simulink model "State_Feedback_Osservatore_Integratore_R"  (R2024b)
settings: Solver=VariableStepAuto  StartTime=0.0  StopTime=ST  RelTol=1e-3
InitFcn:
  | % clear all
  | % close all
  | % clc
  | %
  | % % Load Modello e Parametri
  | % load("model.mat");
  | %
  | % load("Ass_autovalori.mat");
  | %
  | % double_A = double(A_lin);
  | % double_B = double(B_lin);
  | % C = [1 0 0 0 0 0; 0 0 1 0 0 0; 0 0 0 0 1 0];
  | % D = zeros(3,2);
  | % Kf = pinv(C*inv(A_closed_loop)*double_B);
  | %
  | % % Condizioni iniziali
  | % x0 = [1, 0, 0.44, 0, 0.03, 0]'; % Stato iniziale
  | %
  | % % Verifica dell'osservabilità
  | % O = obsv(A_lin, C); rank(O)
  | % osservabile = rank(O) == size(double_A, 1);
  | %
  | % if osservabile
  | %     disp('Il sistema è osservabile.');
  | % else
  | %     disp('Il sistema NON è osservabile.');
  | % end
  | %
  | % % Verifica dell'osservabilità
  | % Ctrb = ctrb(double_A', C');
  | % controllabile = rank(Ctrb) == size(double_A, 1);
  | %
  | % if controllabile
  | %     disp('Il sistema è controllabile.');
  | % else
  | %     disp('Il sistema NON è controllabile.');
  | % end
  | %
  | %
  | % % Poli desiderati per l'osservatore
  | % poli_osservatore = [-80 -2 -40 -1 -30 -0.5];
  | %
  | % % Calcolo del guadagno dell'osservatore L
  | % L = place(double_A', C', poli_osservatore)';
  | %
  | % % Dinamica dell'osservatore
  | % A_o = double_A - L * C; % Matrice del sistema osservatore
  | % B_o = [double_B - L * D, L]; % Matrice degli ingressi per l'osservatore
  | % C_o = eye(6); % Gli stati stimati vengono restituiti
  | % D_o = zeros(6,5); % Dimensioni appropriate per ingressi e uscite
undefined symbols (not defined in the file or in its folder): A_o, B_o, C, C_o, D, D_o, double_A, double_B, K_i, x0, x0_Aug, xd_aug
libraries: simulink x1
settings Model: Creator=raffa  LastModifiedBy=raffa
settings RTWCC: GPUComputeCapability=3.5

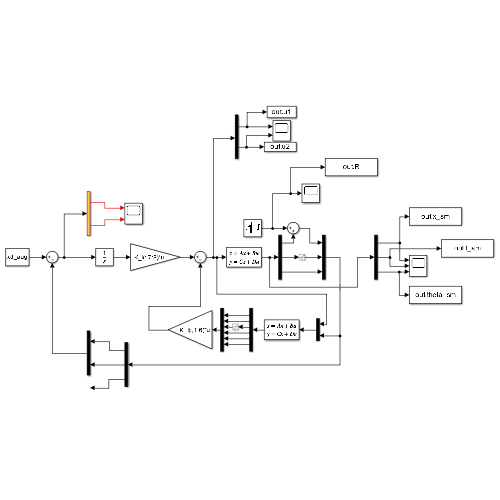
[thumbnail: Simulink's stored preview of the top-level diagram]
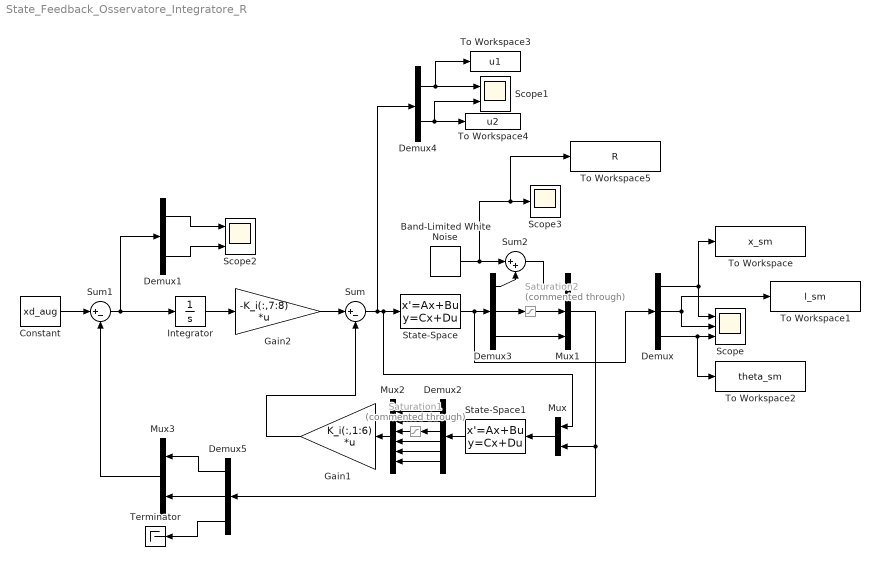
== system State_Feedback_Osservatore_Integratore_R ==
  Band-Limited White Noise : simulink/Sources/Band-Limited White Noise  Cov=[0.00005]  Ts=0.1  seed=[23341]
  Constant : Constant  Value=xd_aug
  Demux : Demux  Outputs=3
  Demux1 : Demux  Outputs=2
  Demux2 : Demux  Outputs=6
  Demux3 : Demux  Outputs=3
  Demux4 : Demux  Outputs=2
  Demux5 : Demux  Outputs=3
  Gain1 : Gain  Gain=K_i(:,1:6)  Multiplication=Matrix(K*u)
  Gain2 : Gain  Gain=-K_i(:,7:8)  Multiplication=Matrix(K*u)
  Integrator : Integrator  InitialCondition="[1 0 0 0 0 0 0 0; 0 0  1 0 0 0 0 0] * x0_Aug"
  Mux : Mux  Inputs=2
  Mux1 : Mux  Inputs=3
  Mux2 : Mux  Inputs=6
  Mux3 : Mux  Inputs=2
  Saturation1 : Saturate  Commented=through  UpperLimit=2  LowerLimit=0.1
  Saturation2 : Saturate  Commented=through  UpperLimit=2  LowerLimit=0.1
  Scope : Scope  NumInputPorts=3
  Scope1 : Scope  NumInputPorts=2
  Scope2 : Scope  NumInputPorts=2
  Scope3 : Scope
  State-Space : StateSpace  A=double_A  B=double_B  C=C  D=D  InitialCondition=x0
  State-Space1 : StateSpace  A=A_o  B=B_o  C=C_o  D=D_o  InitialCondition=x0
  Sum : Sum  Inputs=|+-
  Sum1 : Sum  Inputs=|+-
  Sum2 : Sum  Inputs=|++
  Terminator : Terminator
  To Workspace : ToWorkspace  VariableName=x_sm  SaveFormat=Timeseries  SampleTime=-1
  To Workspace1 : ToWorkspace  VariableName=l_sm  SaveFormat=Timeseries  SampleTime=-1
  To Workspace2 : ToWorkspace  VariableName=theta_sm  SaveFormat=Timeseries  SampleTime=-1
  To Workspace3 : ToWorkspace  VariableName=u1  SaveFormat=Timeseries  SampleTime=-1
  To Workspace4 : ToWorkspace  VariableName=u2  SaveFormat=Timeseries  SampleTime=-1
  To Workspace5 : ToWorkspace  VariableName=R  SaveFormat=Timeseries  SampleTime=-1
  wires:
  Mux1/1 -> Demux5/1, Mux/2
  Gain1/1 -> Sum/2
  Demux/1 -> Scope/1, To Workspace/1
  Demux/2 -> Scope/2, To Workspace1/1
  Mux/1 -> State-Space1/1
  Integrator/1 -> Gain2/1
  Constant/1 -> Sum1/1
  Gain2/1 -> Sum/1
  Sum1/1 -> Integrator/1, Demux1/1
  Demux1/1 -> Scope2/1
  Demux2/1 -> Mux2/1
  Demux2/2 -> Mux2/2
  State-Space1/1 -> Demux2/1
  Mux2/1 -> Gain1/1
  Demux3/2 -> Saturation2/1
  State-Space/1 -> Demux/1, Demux3/1
  Demux4/1 -> To Workspace3/1, Scope1/1
  Sum/1 -> Mux/1, State-Space/1, Demux4/1
  Demux4/2 -> Scope1/2, To Workspace4/1
  Sum2/1 -> Mux1/1
  Demux3/1 -> Sum2/2
  Band-Limited White Noise/1 -> To Workspace5/1, Scope3/1, Sum2/1
  Demux2/4 -> Mux2/4
  Demux2/5 -> Mux2/5
  Demux2/6 -> Mux2/6
  Demux1/2 -> Scope2/2
  Demux3/3 -> Mux1/3
  Demux/3 -> To Workspace2/1, Scope/3
  Demux5/1 -> Mux3/1
  Demux5/2 -> Mux3/2
  Demux5/3 -> Terminator/1
  Mux3/1 -> Sum1/2
  Demux2/3 -> Saturation1/1
  Saturation1/1 -> Mux2/3
  Saturation2/1 -> Mux1/2
